simulink subsystem "LaserMm"  (R2023b)
settings: Solver=VariableStepAuto  StartTime=0.0  StopTime=10.0  RelTol=1e-3
settings Model: Creator=migue  LastModifiedBy=Manuel

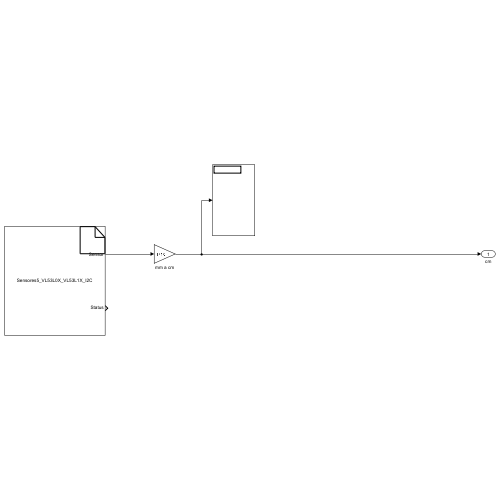
[thumbnail: Simulink's stored preview of the top-level diagram]
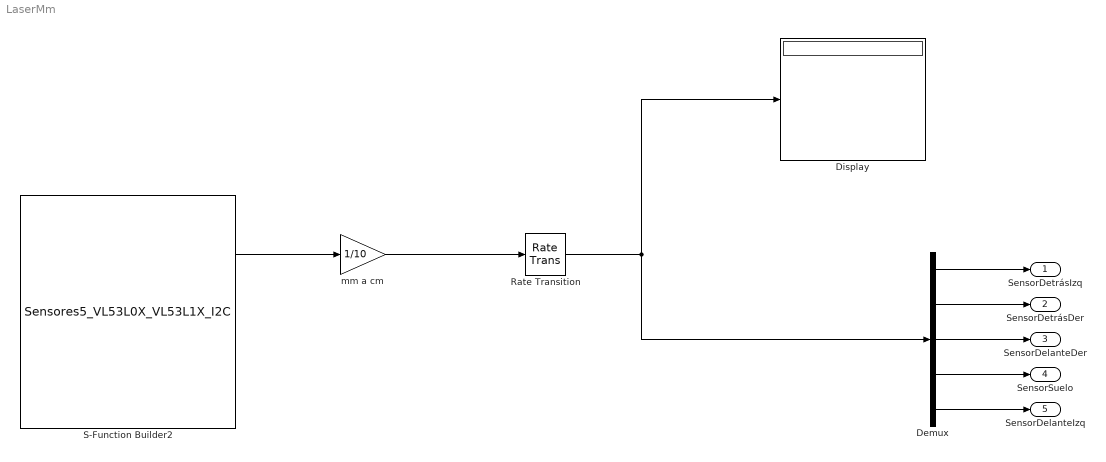
== system LaserMm ==
  Demux : Demux  Outputs=5
  Display : Display
  Rate Transition : RateTransition
  S-Function Builder2 : S-Function  InitFcn=try, set_param(gcb,'FunctionName','Sensores5_VL53L0X_VL53L1X_I2C'), end  FunctionName=Sensores5_VL53L0X_VL53L1X_I2C  SFunctionModules=Sensores5_VL53L0X_VL53L1X_I2C_wrapper.cpp  SFunctionDeploymentMode=off  EnableBusSupport=off  mask(S-Function Builder){}
      mask help: Simulink:masks:SFunctionBuilder_MD
      mask init:
      | val = [[.9  0.75 0.75 1 1 .9 .9 1]',[1 1 0.75 0.75 .9 .9 1 .9]'];try , sys = get_param(gcb,'SfunBuilderFcnName');if isempty(sys), sys = get_param(gcb,'FunctionName'); end,catch, sys = get_param(gcb,'FunctionName'); end
      settings: CopyFcn=set_param(gcbh,'LinkStatus','none')  PreSaveFcn=try, set_param(gcb,'FunctionName','Sensores5_VL53L0X_VL53L1X_I2C'), end  OpenFcn=sfunctionwizard(gcbh)
      mask Display:
      | plot(val(:,1),val(:,2))
      | disp(sys)
      | port_label('output',1,'Sensor')
      | port_label('output',2,'Status')
  mm a cm : Gain  Gain=1/10
  SensorDetrásIzq : Outport
  SensorDetrásDer : Outport  Port=2
  SensorDelanteDer : Outport  Port=3
  SensorSuelo : Outport  Port=4
  SensorDelanteIzq : Outport  Port=5
  wires:
  S-Function Builder2/1 -> mm a cm/1
  mm a cm/1 -> Rate Transition/1
  Rate Transition/1 -> Display/1, Demux/1
  Demux/1 -> SensorDetrásIzq/1
  Demux/2 -> SensorDetrásDer/1
  Demux/3 -> SensorDelanteDer/1
  Demux/4 -> SensorSuelo/1
  Demux/5 -> SensorDelanteIzq/1
